simulink subsystem "distance_sensor"  (R2022b)
settings: Solver=VariableStepAuto  StartTime=0.0  StopTime=10.0  RelTol=1e-3
model mask{Pin=A0, Breakpoints=[], Table=[]}
  mask prompts: Pin "svd:svd:PinPrompt"; Table "Simulink:blkprm_prompts:InterpndTable"
libraries: mbedblockslib x1, dspstat3 x1
settings Model: Creator=micha  LastModifiedBy=micha

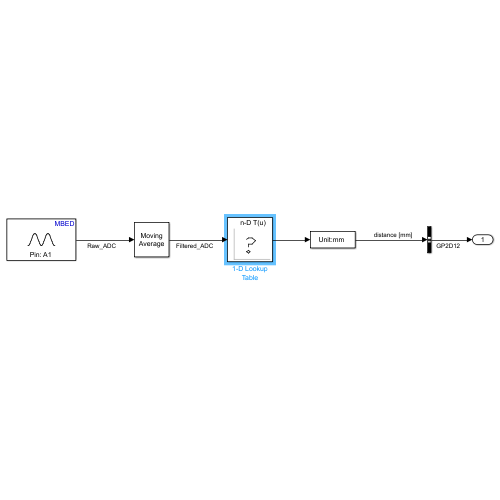
[thumbnail: Simulink's stored preview of the top-level diagram]
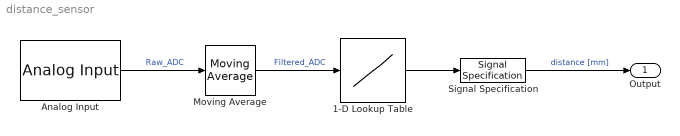
== system distance_sensor ==
  1-D Lookup Table : Lookup_n-D  NumberOfTableDimensions=1  BreakpointsForDimension1=Breakpoints  Table=Table  InternalRulePriority=Speed  RndMeth=Simplest
  Analog Input : mbedblockslib/Analog Input  Pin=A2  ReadResultsOnly=off  ConversionTriggerSource=Software  ExternalTriggerType=uint32( 0 )  OutputDataType=double  EnableConversionCompleteNotify=off  EnableOuputStatus=off  SampleTime=-1
      settings: LibrarySourceBlock=stmnucleorootlib/Common/Analog Input
  Moving Average : dspstat3/Moving Average  Method=Sliding window  ForgettingFactorPort=off  SpecifyWindowLength=on  WindowLength=20  OverlapLength=19  AllowArbitraryInputLength=off  ForgettingFactor=0.9  SimulateUsing=Code generation
  Signal Specification : SignalSpecification  Unit=mm
  Output : Outport
  wires:
  Moving Average/1 -> 1-D Lookup Table/1  "Filtered_ADC"
  Signal Specification/1 -> Output/1  "distance [mm]"
  1-D Lookup Table/1 -> Signal Specification/1
  Analog Input/1 -> Moving Average/1  "Raw_ADC"
